simulink model "Lab7_Digital"  (R2012b)
settings: Solver=ode45  StartTime=0.0  StopTime=250  RelTol=1e-3
values from neighbouring files (symbols this model uses):
  T = 1    [Lab7_Discrete.m]
undefined symbols (not defined in the file or in its folder): dD, nD
settings Model: Creator=Viktor  LastModifiedBy=Viktor

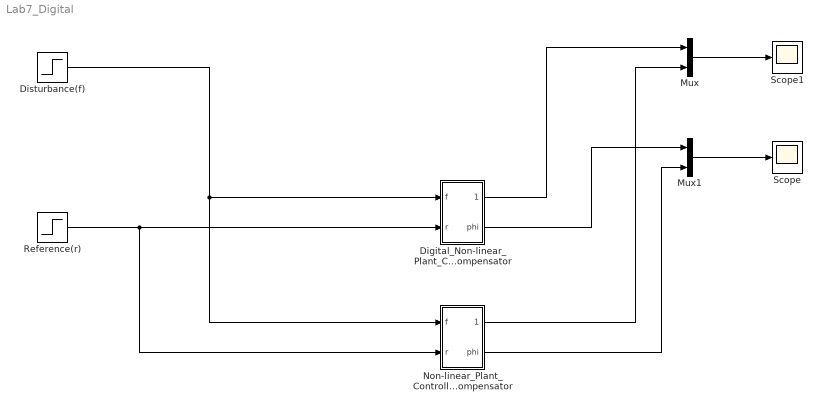
== system Lab7_Digital ==
  Digital_Non-linear_Plant_Controller_Anti_Windup_Compensator : Subsystem
  Disturbance(f) : Step  Time=0  After=2  SampleTime=0
  Mux : Mux  Inputs=2
  Mux1 : Mux  Inputs=2
  Non-linear_Plant_Controller_Anti_Windup_Compensator : Subsystem
  Reference(r) : Step  Time=0  After=30  SampleTime=0
  Scope : Scope
  Scope1 : Scope
  wires:
  Digital_Non-linear_Plant_Controller_Anti_Windup_Compensator/2(phi) -> Mux1/1
  Digital_Non-linear_Plant_Controller_Anti_Windup_Compensator/1(delta) -> Mux/1
  Disturbance(f)/1 -> Digital_Non-linear_Plant_Controller_Anti_Windup_Compensator/1(f), Non-linear_Plant_Controller_Anti_Windup_Compensator/1(f)
  Reference(r)/1 -> Digital_Non-linear_Plant_Controller_Anti_Windup_Compensator/2(r), Non-linear_Plant_Controller_Anti_Windup_Compensator/2(r)
  Non-linear_Plant_Controller_Anti_Windup_Compensator/2(phi) -> Mux1/2
  Non-linear_Plant_Controller_Anti_Windup_Compensator/1(delta) -> Mux/2
  Mux/1 -> Scope1/1
  Mux1/1 -> Scope/1

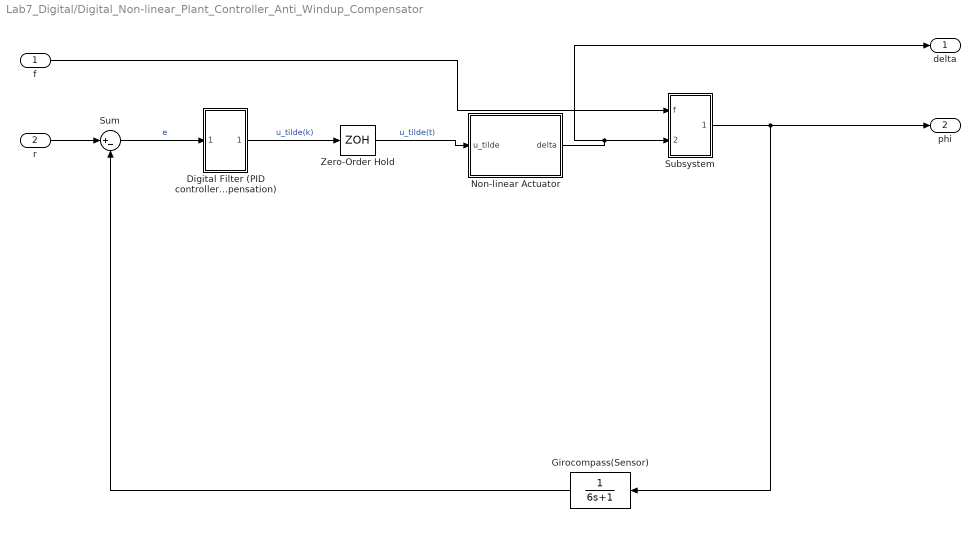
== system Lab7_Digital/Digital_Non-linear_Plant_Controller_Anti_Windup_Compensator ==
  f : Inport
  r : Inport  Port=2
  Digital Filter (PID controller wind-up compensation) : Subsystem
  Girocompass(Sensor) : TransferFcn  Denominator=[6 1]
  Non-linear Actuator : Subsystem
  Subsystem : Subsystem
  Sum : Sum  Inputs=|+-
  Zero-Order Hold : ZeroOrderHold  SampleTime=T
  delta : Outport
  phi : Outport  Port=2
  wires:
  Subsystem/1(phi) -> Girocompass(Sensor)/1, phi/1
  f/1 -> Subsystem/1("f ")
  Girocompass(Sensor)/1 -> Sum/2
  r/1 -> Sum/1
  Non-linear Actuator/1(delta) -> delta/1, Subsystem/2(delta)
  Sum/1 -> Digital Filter (PID controller wind-up compensation)/1(In1)  "e"
  Digital Filter (PID controller wind-up compensation)/1(Out1) -> Zero-Order Hold/1  "u_tilde(k)"
  Zero-Order Hold/1 -> Non-linear Actuator/1(u_tilde)  "u_tilde(t)"

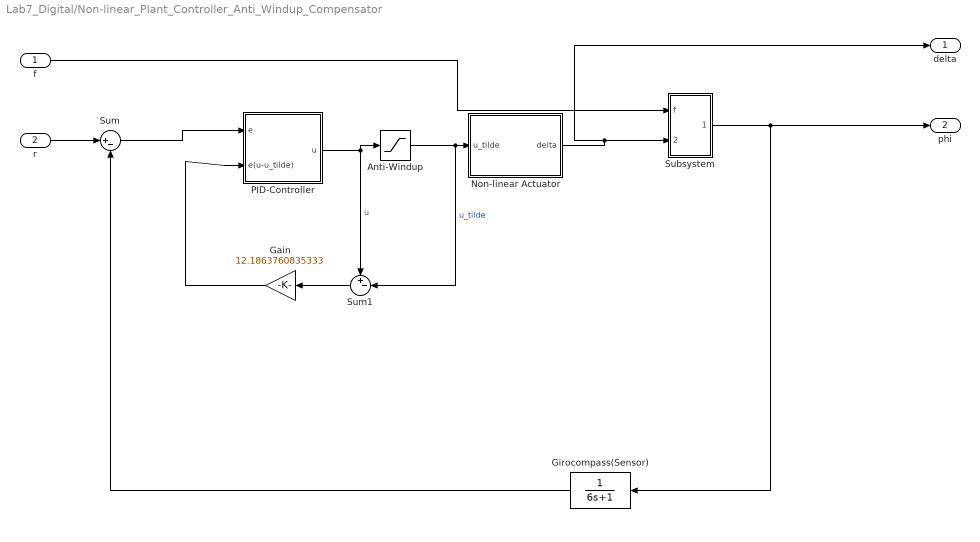
== system Lab7_Digital/Non-linear_Plant_Controller_Anti_Windup_Compensator ==
  f : Inport
  r : Inport  Port=2
  Anti-Windup : Saturate  UpperLimit=30  LowerLimit=-30
  Gain : Gain  Gain=12.1863760835333
  Girocompass(Sensor) : TransferFcn  Denominator=[6 1]
  Non-linear Actuator : Subsystem
  PID-Controller : Subsystem
  Subsystem : Subsystem
  Sum : Sum  Inputs=|+-
  Sum1 : Sum  Inputs=+-|
  delta : Outport
  phi : Outport  Port=2
  wires:
  Subsystem/1(phi) -> Girocompass(Sensor)/1, phi/1
  f/1 -> Subsystem/1("f ")
  Sum/1 -> PID-Controller/1(e)
  Girocompass(Sensor)/1 -> Sum/2
  r/1 -> Sum/1
  Non-linear Actuator/1(delta) -> delta/1, Subsystem/2(delta)
  PID-Controller/1(u) -> Sum1/1, Anti-Windup/1  "u"
  Anti-Windup/1 -> Sum1/2, Non-linear Actuator/1(u_tilde)  "u_tilde"
  Sum1/1 -> Gain/1
  Gain/1 -> PID-Controller/2(e(u-u_tilde))

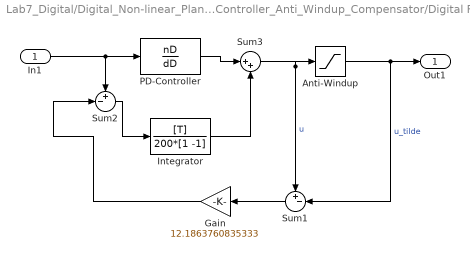
== system Lab7_Digital/Digital_Non-linear_Plant_Controller_Anti_Windup_Compensator/Digital Filter (PID controller wind-up compensation) ==
  In1 : Inport
  Anti-Windup : Saturate  UpperLimit=30  LowerLimit=-30
  Gain : Gain  Gain=12.1863760835333
  Integrator : DiscreteTransferFcn  Numerator=[T]  Denominator=200*[1 -1]  SampleTime=T
  PD-Controller : DiscreteTransferFcn  Numerator=nD  Denominator=dD  SampleTime=T
  Sum1 : Sum  Inputs=+-|
  Sum2 : Sum  Inputs=+-|
  Sum3 : Sum  Inputs=|++
  Out1 : Outport
  wires:
  PD-Controller/1 -> Sum3/1
  Integrator/1 -> Sum3/2
  Sum2/1 -> Integrator/1
  Gain/1 -> Sum2/2
  Sum1/1 -> Gain/1
  Anti-Windup/1 -> Out1/1, Sum1/2  "u_tilde"
  Sum3/1 -> Sum1/1, Anti-Windup/1  "u"
  In1/1 -> Sum2/1, PD-Controller/1

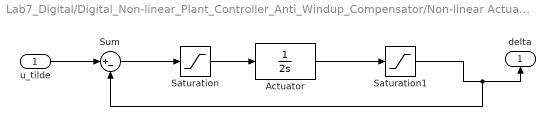
== system Lab7_Digital/Digital_Non-linear_Plant_Controller_Anti_Windup_Compensator/Non-linear Actuator ==
  u_tilde : Inport
  Actuator : TransferFcn  Denominator=[2 0]
  Saturation : Saturate  UpperLimit=3  LowerLimit=-3
  Saturation1 : Saturate  UpperLimit=30  LowerLimit=-30
  Sum : Sum  Inputs=|+-
  delta : Outport
  wires:
  u_tilde/1 -> Sum/1
  Sum/1 -> Saturation/1
  Saturation/1 -> Actuator/1
  Actuator/1 -> Saturation1/1
  Saturation1/1 -> Sum/2, delta/1

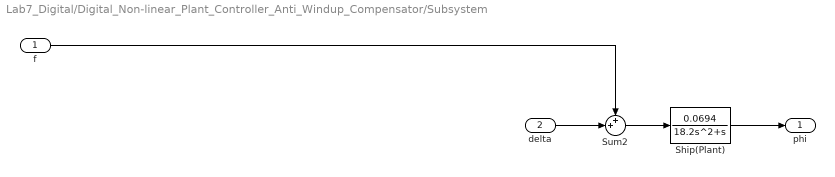
== system Lab7_Digital/Digital_Non-linear_Plant_Controller_Anti_Windup_Compensator/Subsystem ==
  "f " : Inport
  delta : Inport  Port=2
  Ship(Plant) : TransferFcn  Numerator=[0.0694]  Denominator=[18.2 1 0]
  Sum2 : Sum  Inputs=++|
  phi : Outport
  wires:
  delta/1 -> Sum2/2
  "f "/1 -> Sum2/1
  Sum2/1 -> Ship(Plant)/1
  Ship(Plant)/1 -> phi/1

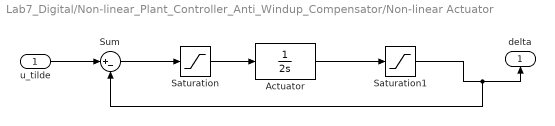
== system Lab7_Digital/Non-linear_Plant_Controller_Anti_Windup_Compensator/Non-linear Actuator ==
  u_tilde : Inport
  Actuator : TransferFcn  Denominator=[2 0]
  Saturation : Saturate  UpperLimit=3  LowerLimit=-3
  Saturation1 : Saturate  UpperLimit=30  LowerLimit=-30
  Sum : Sum  Inputs=|+-
  delta : Outport
  wires:
  u_tilde/1 -> Sum/1
  Sum/1 -> Saturation/1
  Saturation/1 -> Actuator/1
  Actuator/1 -> Saturation1/1
  Saturation1/1 -> Sum/2, delta/1

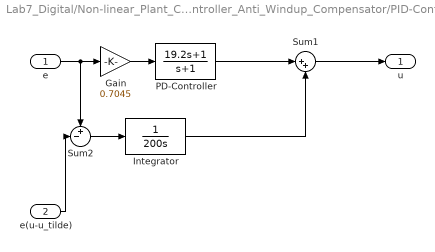
== system Lab7_Digital/Non-linear_Plant_Controller_Anti_Windup_Compensator/PID-Controller ==
  e : Inport
  e(u-u_tilde) : Inport  Port=2
  Gain : Gain  Gain=0.7045
  Integrator : TransferFcn  Denominator=[200 0]
  PD-Controller : TransferFcn  Numerator=[19.2 1]  Denominator=[1 1]
  Sum1 : Sum  Inputs=|++
  Sum2 : Sum  Inputs=+-|
  u : Outport
  wires:
  Integrator/1 -> Sum1/2
  PD-Controller/1 -> Sum1/1
  e/1 -> Sum2/1, Gain/1
  Gain/1 -> PD-Controller/1
  Sum1/1 -> u/1
  Sum2/1 -> Integrator/1
  e(u-u_tilde)/1 -> Sum2/2

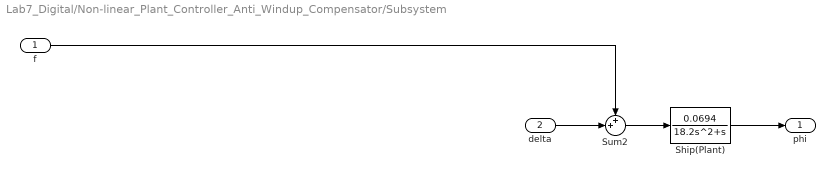
== system Lab7_Digital/Non-linear_Plant_Controller_Anti_Windup_Compensator/Subsystem ==
  "f " : Inport
  delta : Inport  Port=2
  Ship(Plant) : TransferFcn  Numerator=[0.0694]  Denominator=[18.2 1 0]
  Sum2 : Sum  Inputs=++|
  phi : Outport
  wires:
  delta/1 -> Sum2/2
  "f "/1 -> Sum2/1
  Sum2/1 -> Ship(Plant)/1
  Ship(Plant)/1 -> phi/1
